simulink model "NCKH"  (R2016a)
settings: Solver=ode5  StartTime=0.0  StopTime=inf  FixedStep=0.05  RelTol=1e-3
InitFcn:
  | ts=0.05;
values from neighbouring files (symbols this model uses):
  deta = [0.0523598775598 0.0644817894383 0.076588183533 0.0886635951506 0.10069266521 0.112660191642 0.124551179125 0.136350886659 0.148044872522 0.159619036175 0.171059656781 0.199806720549 ... (2400 elements, 200x12)]    [deta.mat]
libraries: arduinolib x12
settings Model: SimulationMode=external  ExtModeTrigDuration=2  Creator=ACER  LastModifiedBy=ACER
settings OptimizationCC: OptimizeModelRefInitCode=on  LifeSpan=Inf  MaxStackSize=64
settings HardwareCC: ProdBitPerPointer=32  ProdLargestAtomicInteger=Long  ProdLargestAtomicFloat=Double  ProdWordSize=32  ProdHWDeviceType=ARM Compatible->ARM Cortex
settings RTWCC: SystemTargetFile=ert.tlc  HardwareBoard=Arduino Due  TemplateMakefile=ert_default_tmf  GenerateReport=on  Toolchain=Arduino ARM v1.6.1  BuildConfiguration=Faster Runs  IncludeHyperlinkInReport=on  LaunchReport=on  GenerateTraceInfo=on  GenerateTraceReport=on  GenerateTraceReportSl=on  GenerateTraceReportSf=on  GenerateTraceReportEml=on
settings CodeAppCC: ForceParamTrailComments=on  IgnoreCustomStorageClasses=off  OperatorAnnotations=on  SimulinkDataObjDesc=on  SFDataObjDesc=on  MATLABFcnDesc=on  InsertBlockDesc=on  MATLABSourceComments=on
settings ERTTargetCC: SupportContinuousTime=on  SupportVariableSizeSignals=on

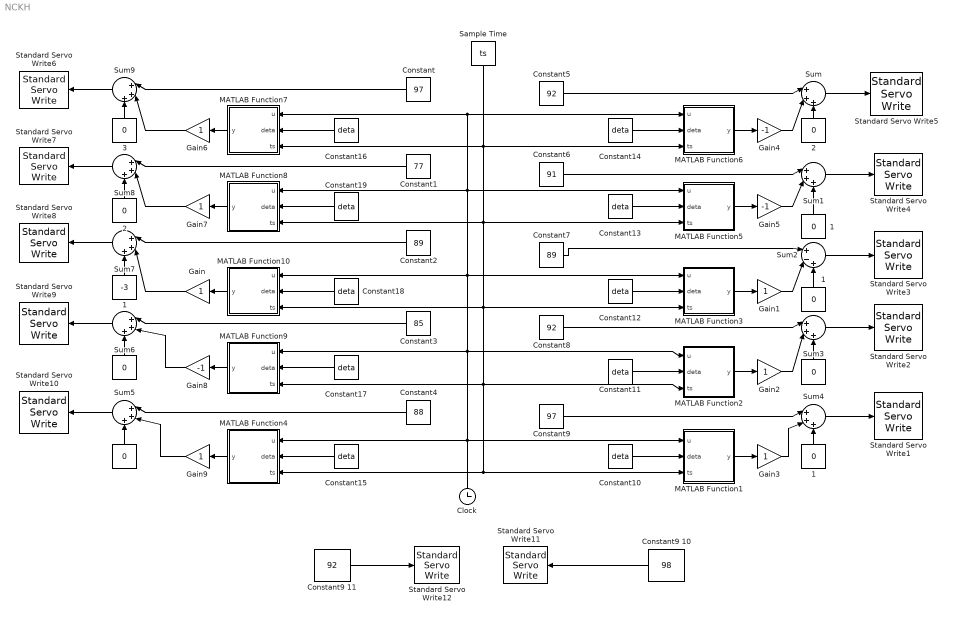
== system NCKH ==
   {,,,1,1,1..2,2..3} (9 alike) : Constant  Value=0
  " 1" : Constant  Value=-3
  Clock : Clock
  Constant : Constant  Value=97
  Constant1 : Constant  Value=77
  Constant{10..19} (10 alike) : Constant  Value=deta
  Constant2 : Constant  Value=89
  Constant3 : Constant  Value=85
  Constant4 : Constant  Value=88
  Constant5 : Constant  Value=92
  Constant6 : Constant  Value=91
  Constant7 : Constant  Value=89
  Constant8 : Constant  Value=92
  Constant9 : Constant  Value=97
  Constant9 10 : Constant  Value=98
  Constant9 11 : Constant  Value=92
  Gain{,1..3,6..7,9} (7 alike) : Gain
  Gain4 : Gain  Gain=-1
  Gain5 : Gain  Gain=-1
  Gain8 : Gain  Gain=-1
  MATLAB Function1 : MATLAB Function  TreatAsAtomicUnit=on
  MATLAB Function10 : MATLAB Function  TreatAsAtomicUnit=on
  MATLAB Function2 : MATLAB Function  TreatAsAtomicUnit=on
  MATLAB Function3 : MATLAB Function  TreatAsAtomicUnit=on
  MATLAB Function4 : MATLAB Function  TreatAsAtomicUnit=on
  MATLAB Function5 : MATLAB Function  TreatAsAtomicUnit=on
  MATLAB Function6 : MATLAB Function  TreatAsAtomicUnit=on
  MATLAB Function7 : MATLAB Function  TreatAsAtomicUnit=on
  MATLAB Function8 : MATLAB Function  TreatAsAtomicUnit=on
  MATLAB Function9 : MATLAB Function  TreatAsAtomicUnit=on
  Sample Time : Constant  Value=ts  SampleTime=0.05
  Standard Servo Write1 : arduinolib/Standard Servo Write  pinNumber=2  blockPlatform=arduino
  Standard Servo Write10 : arduinolib/Standard Servo Write  pinNumber=11  blockPlatform=arduino
  Standard Servo Write11 : arduinolib/Standard Servo Write  pinNumber=12  blockPlatform=arduino
  Standard Servo Write12 : arduinolib/Standard Servo Write  pinNumber=13  blockPlatform=arduino
  Standard Servo Write2 : arduinolib/Standard Servo Write  pinNumber=3  blockPlatform=arduino
  Standard Servo Write3 : arduinolib/Standard Servo Write  pinNumber=4  blockPlatform=arduino
  Standard Servo Write4 : arduinolib/Standard Servo Write  pinNumber=5  blockPlatform=arduino
  Standard Servo Write5 : arduinolib/Standard Servo Write  pinNumber=6  blockPlatform=arduino
  Standard Servo Write6 : arduinolib/Standard Servo Write  pinNumber=7  blockPlatform=arduino
  Standard Servo Write7 : arduinolib/Standard Servo Write  pinNumber=8  blockPlatform=arduino
  Standard Servo Write8 : arduinolib/Standard Servo Write  pinNumber=9  blockPlatform=arduino
  Standard Servo Write9 : arduinolib/Standard Servo Write  pinNumber=10  blockPlatform=arduino
  Sum{,1,3..9} (9 alike) : Sum  Inputs=|+++
  Sum2 : Sum  Inputs=|+-+
  wires:
  Sum/1 -> Standard Servo Write5/1
  Sum1/1 -> Standard Servo Write4/1
  Sum2/1 -> Standard Servo Write3/1
  Sum3/1 -> Standard Servo Write2/1
  Sum4/1 -> Standard Servo Write1/1
  Sum5/1 -> Standard Servo Write10/1
  Sum6/1 -> Standard Servo Write9/1
  Sum7/1 -> Standard Servo Write8/1
  Sum8/1 -> Standard Servo Write7/1
  Sum9/1 -> Standard Servo Write6/1
  MATLAB Function7/1(y) -> Gain6/1
  MATLAB Function8/1(y) -> Gain7/1
  MATLAB Function9/1(y) -> Gain8/1
  MATLAB Function4/1(y) -> Gain9/1
  MATLAB Function2/1(y) -> Gain2/1
  MATLAB Function1/1(y) -> Gain3/1
  MATLAB Function5/1(y) -> Gain5/1
  MATLAB Function6/1(y) -> Gain4/1
  Constant/1 -> Sum9/1
  Constant1/1 -> Sum8/1
  Constant3/1 -> Sum6/1
  Constant4/1 -> Sum5/1
  Constant2/1 -> Sum7/1
  Constant5/1 -> Sum/1
  Constant9/1 -> Sum4/1
  Constant8/1 -> Sum3/1
  Constant7/1 -> Sum2/1
  Constant6/1 -> Sum1/1
  Gain/1 -> Sum7/2
  MATLAB Function10/1(y) -> Gain/1
  MATLAB Function3/1(y) -> Gain1/1
  Gain1/1 -> Sum2/2
  Constant10/1 -> MATLAB Function1/2(deta)
  Constant11/1 -> MATLAB Function2/2(deta)
  Constant12/1 -> MATLAB Function3/2(deta)
  Constant13/1 -> MATLAB Function5/2(deta)
  Constant14/1 -> MATLAB Function6/2(deta)
  Constant16/1 -> MATLAB Function7/2(deta)
  Clock/1 -> MATLAB Function1/1(u), MATLAB Function10/1(u), MATLAB Function5/1(u), MATLAB Function7/1(u), MATLAB Function6/1(u), MATLAB Function8/1(u), MATLAB Function3/1(u), MATLAB Function2/1(u), MATLAB Function9/1(u), MATLAB Function4/1(u)
  Constant17/1 -> MATLAB Function9/2(deta)
  Constant18/1 -> MATLAB Function10/2(deta)
  Constant19/1 -> MATLAB Function8/2(deta)
  Sample Time/1 -> MATLAB Function8/3(ts), MATLAB Function10/3(ts), MATLAB Function3/3(ts), MATLAB Function4/3(ts), MATLAB Function1/3(ts), MATLAB Function2/3(ts), MATLAB Function9/3(ts), MATLAB Function5/3(ts), MATLAB Function7/3(ts), MATLAB Function6/3(ts)
  Gain5/1 -> Sum1/2
  Gain2/1 -> Sum3/2
  Gain3/1 -> Sum4/2
  Gain4/1 -> Sum/2
  Gain6/1 -> Sum9/2
  Gain7/1 -> Sum8/2
  Gain8/1 -> Sum6/2
  Gain9/1 -> Sum5/2
  " "/1 -> Sum5/3
  " "/1 -> Sum3/3
  " 1"/1 -> Sum1/3
  " 1"/1 -> Sum4/3
  " 1"/1 -> Sum7/3
  " 2"/1 -> Sum8/3
  " 3"/1 -> Sum9/3
  " 2"/1 -> Sum/3
  Constant15/1 -> MATLAB Function4/2(deta)
  " 1"/1 -> Sum2/3
  Constant9 10/1 -> Standard Servo Write11/1
  Constant9 11/1 -> Standard Servo Write12/1
  " "/1 -> Sum6/3

== matlab function NCKH/MATLAB Function2 ==
  data: u input; y output; deta input; ts input
function y = fcn(u,deta,ts)
%#codegen
Deta2 = deta(:,2)*180/pi;
k = mod(round(u/ts), 200)+1;
y=Deta2(k);

== matlab function NCKH/MATLAB Function1 ==
  data: u input; y output; deta input; ts input
function y = fcn(u,deta,ts)
%#codegen
Deta1 = deta(:,1)*180/pi;
k = mod(round(u/ts), 200)+1;  
y = Deta1(k);

== matlab function NCKH/MATLAB Function3 ==
  data: u input; y output; deta input; ts input
function y = fcn(u,deta,ts)
%#codegen
Deta3 = deta(:,3)*180/pi;
k = mod(round(u/ts), 200)+1;
y=Deta3(k);

== matlab function NCKH/MATLAB Function5 ==
  data: u input; y output; deta input; ts input
function y = fcn(u,deta,ts)
%#codegen
Deta5 = deta(:,5)*180/pi;
k = mod(round(u/ts), 200)+1;
y=Deta5(k);

== matlab function NCKH/MATLAB Function6 ==
  data: u input; y output; deta input; ts input
function y = fcn(u,deta,ts)
%#codegen
Deta6 = deta(:,6)*180/pi;
k = mod(round(u/ts), 200)+1;
y=Deta6(k);

== matlab function NCKH/MATLAB Function7 ==
  data: u input; y output; deta input; ts input
function y = fcn(u,deta,ts)
%#codegen 
Deta7 = deta(:,7)*180/pi;    
k = mod(round(u/ts), 200)+1;
y=Deta7(k);

== matlab function NCKH/MATLAB Function8 ==
  data: u input; y output; deta input; ts input
function y = fcn(u,deta,ts)
%#codegen
Deta8 = deta(:,8)*180/pi;
k = mod(round(u/ts),200)+1;
y=Deta8(k);

== matlab function NCKH/MATLAB Function10 ==
  data: u input; y output; deta input; ts input
function y = fcn(u,deta,ts)
%#codegen
Deta10 = deta(:,10)*180/pi;
k = mod(round(u/ts), 200)+1;
y=Deta10(k);

== matlab function NCKH/MATLAB Function9 ==
  data: u input; y output; deta input; ts input
function y = fcn(u,deta,ts)
%#codegen
Deta11 = deta(:,11)*180/pi;
k = mod(round(u/ts), 200)+1;
y=Deta11(k);

== matlab function NCKH/MATLAB Function4 ==
  data: u input; y output; deta input; ts input
function y = fcn(u,deta,ts)
%#codegen
Deta12 = deta(:,12)*180/pi;
k = mod(round(u/ts), 200)+1;  
y = Deta12(k);
